simulink model "Charge_Pumps_Rev0"  (R2019b)
settings: Solver=VariableStepAuto  StartTime=0.0  StopTime=0.3e-3  RelTol=1e-3
libraries: simulink x4, simulink_extras x1
settings Model: Creator=connerhannon  LastModifiedBy=connerhannon

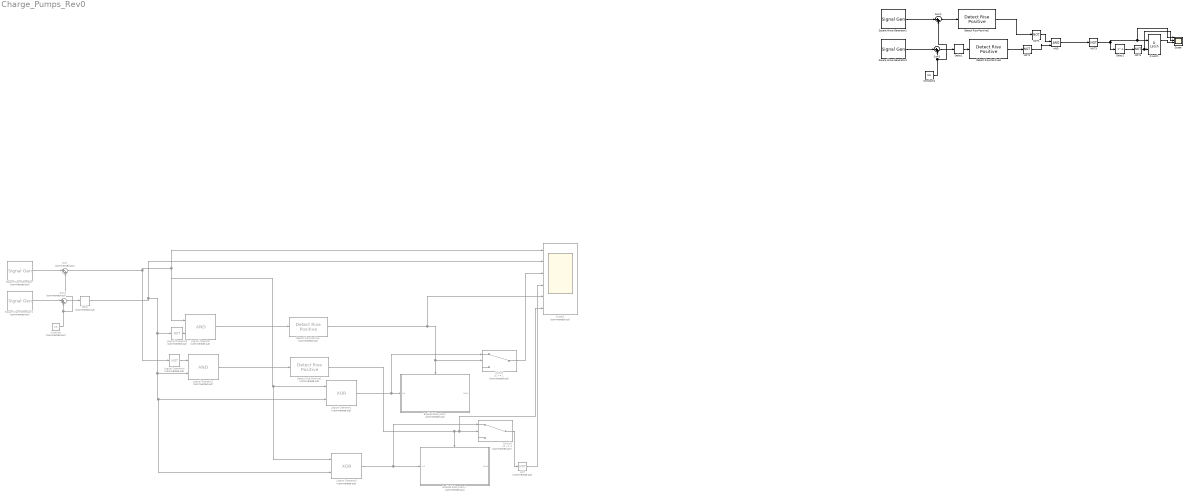
== system Charge_Pumps_Rev0 ==
  AND : Logic  IconShape=distinctive  AllPortsSameDT=off  OutDataTypeStr=boolean
  Constant : Constant  Commented=on  Value=0.5
  Constant1 : Constant  Value=0.5
  D Latch : simulink_extras/Flip Flops/D Latch
      settings: SourceProductName=Simulink  SourceProductBaseCode=SL
  Delay : Delay  Commented=on  DelayLength=2000  InitialCondition=0
  Delay1 : Delay  DelayLength=2000  InitialCondition=0
  Delay2 : Delay  DelayLength=1  InitialCondition=0
  Detect Rise Positive : simulink/Logic and Bit Operations/Detect Rise Positive  Commented=on  vinit=0  OutDataTypeStr=boolean
  Detect Rise Positive1 : simulink/Logic and Bit Operations/Detect Rise Positive  Commented=on  vinit=0  OutDataTypeStr=boolean
  Detect Rise Positive2 : simulink/Logic and Bit Operations/Detect Rise Positive  vinit=0  OutDataTypeStr=boolean
  Detect Rise Positive3 : simulink/Logic and Bit Operations/Detect Rise Positive  vinit=0  OutDataTypeStr=boolean
  Enabled Subsystem : Subsystem  Commented=on  TreatAsAtomicUnit=on
  Enabled Subsystem1 : Subsystem  Commented=on  TreatAsAtomicUnit=on
  Logical Operator : Logic  Commented=on  IconShape=distinctive  AllPortsSameDT=off  OutDataTypeStr=boolean
  Logical Operator1 : Logic  Commented=on  Operator=XOR  IconShape=distinctive  AllPortsSameDT=off  OutDataTypeStr=boolean
  Logical Operator2 : Logic  Commented=on  IconShape=distinctive  AllPortsSameDT=off  OutDataTypeStr=boolean
  Logical Operator3 : Logic  Commented=on  Operator=NOT  IconShape=distinctive  AllPortsSameDT=off  OutDataTypeStr=boolean
  Logical Operator4 : Logic  Commented=on  Operator=NOT  IconShape=distinctive  AllPortsSameDT=off  OutDataTypeStr=boolean
  Logical Operator5 : Logic  Commented=on  Operator=XOR  IconShape=distinctive  AllPortsSameDT=off  OutDataTypeStr=boolean
  NOT : Logic  Commented=on  Operator=NOT  IconShape=distinctive  AllPortsSameDT=off  OutDataTypeStr=boolean
  NOT{1..4} (4 alike) : Logic  Operator=NOT  IconShape=distinctive  AllPortsSameDT=off  OutDataTypeStr=boolean
  Scope : Scope  NumInputPorts=4
  Scope1 : Scope  Commented=on  NumInputPorts=6
  Square Wave Generator : SignalGenerator  Commented=on  WaveForm=square  Amplitude=0.5  Frequency=100000
  Square Wave Generator1 : SignalGenerator  Commented=on  WaveForm=square  Amplitude=0.5  Frequency=100000
  Square Wave Generator2 : SignalGenerator  WaveForm=square  Amplitude=0.5  Frequency=100000
  Square Wave Generator3 : SignalGenerator  WaveForm=square  Amplitude=0.5  Frequency=100000
  Sum : Sum  Commented=on  Inputs=|++
  Sum1 : Sum  Commented=on  Inputs=|++
  Sum2 : Sum  Inputs=|++
  Sum3 : Sum  Inputs=|++
  Switch : Switch  Commented=on  Threshold=1
  Switch1 : Switch  Commented=on  Threshold=1
  wires:
  Logical Operator3/1 -> Logical Operator/2
  Logical Operator4/1 -> Logical Operator2/1
  Logical Operator2/1 -> Detect Rise Positive1/1
  Logical Operator/1 -> Detect Rise Positive/1
  Logical Operator1/1 -> Switch/1, Enabled Subsystem/1(In1)
  Logical Operator5/1 -> Switch1/1, Enabled Subsystem1/1(In1)
  Delay/1 -> Scope1/2, Logical Operator5/2, Logical Operator1/2, Logical Operator2/2, Logical Operator3/1
  NOT/1 -> Scope1/4
  Square Wave Generator/1 -> Sum/1
  Square Wave Generator1/1 -> Sum1/1
  Sum1/1 -> Delay/1
  Constant/1 -> Sum/2, Sum1/2
  Sum/1 -> Scope1/1, Logical Operator5/1, Logical Operator1/1, Logical Operator/1, Logical Operator4/1
  Detect Rise Positive/1 -> Scope1/5, Enabled Subsystem/Enable, Switch/2
  Detect Rise Positive1/1 -> Scope1/6, Switch1/2, Enabled Subsystem1/Enable
  Switch/1 -> Scope1/3
  Switch1/1 -> NOT/1
  Sum3/1 -> Delay1/1
  Constant1/1 -> Sum2/2, Sum3/2
  Square Wave Generator2/1 -> Sum2/1
  Square Wave Generator3/1 -> Sum3/1
  Sum2/1 -> Detect Rise Positive2/1
  Delay1/1 -> Detect Rise Positive3/1
  Detect Rise Positive2/1 -> NOT1/1
  NOT1/1 -> AND/1
  Detect Rise Positive3/1 -> NOT2/1
  AND/1 -> NOT3/1
  NOT2/1 -> AND/2
  NOT3/1 -> Delay2/1, Scope/1, D Latch/1
  NOT4/1 -> Scope/2, D Latch/2
  D Latch/1 -> Scope/3
  Delay2/1 -> NOT4/1

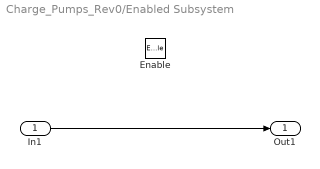
== system Charge_Pumps_Rev0/Enabled Subsystem ==
  In1 : Inport
  Enable : EnablePort  StatesWhenEnabling=reset
  Out1 : Outport
  wires:
  In1/1 -> Out1/1

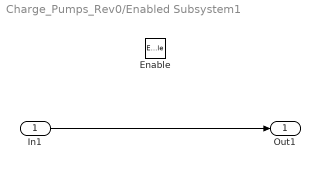
== system Charge_Pumps_Rev0/Enabled Subsystem1 ==
  In1 : Inport
  Enable : EnablePort
  Out1 : Outport
  wires:
  In1/1 -> Out1/1
